simulink model "ADCS_orbiter"  (R2021b)
settings: Solver=VariableStepAuto  StartTime=0.0  StopTime=43200  FixedStep=0.01  MaxStep=1  RelTol=1e-8
values from neighbouring files (symbols this model uses):
  J = [Jx,0,0 ... (first row only)    [Data_detumbling.m]    (also in DisturbanceEvaluation.m = {J_NSO; J_SO}; Thruster_sizing_2.m = diag([12043.36, 15990.19, 8547.84]); main_orbiter.m = J_SO; main_orbiter_detumbling.m = J_SO)
  muE = (6.6743e-11)*(1.0802e20)    (= 7209578860)    [DisturbanceEvaluation.m]    (also in main_orbiter.m; main_orbiter_detumbling.m)
  muS = 3.7931187*1e16    (= 3.7931187e+16)    [DisturbanceEvaluation.m]    (also in main_orbiter.m; main_orbiter_detumbling.m)
  qbn0 = qrand./norm(qrand)    [main_orbiter.m]    (also in main_orbiter_detumbling.m)
  sigma_ARW = deg2rad(0.001)    [main_orbiter_detumbling.m]
  sigma_RRW = deg2rad(0.001)    [main_orbiter_detumbling.m]
  wb0 = 0.0001*rand(3, 1)    [main_orbiter.m]    (also in main_orbiter_detumbling.m = 0.1*rand(3, 1))
  Xpos = reshape(st_pos, [6, 1, L])    [main_orbiter.m]
undefined symbols (not defined in the file or in its folder): ICs, S
libraries: matrix_library x3, sublib_quat x1
settings Model: Creator=pietr  LastModifiedBy=26ele

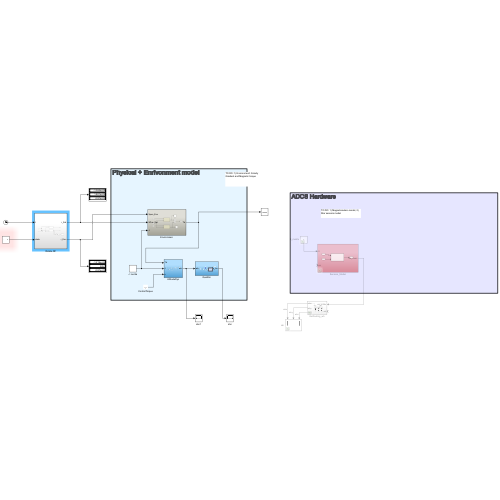
[thumbnail: Simulink's stored preview of the top-level diagram]
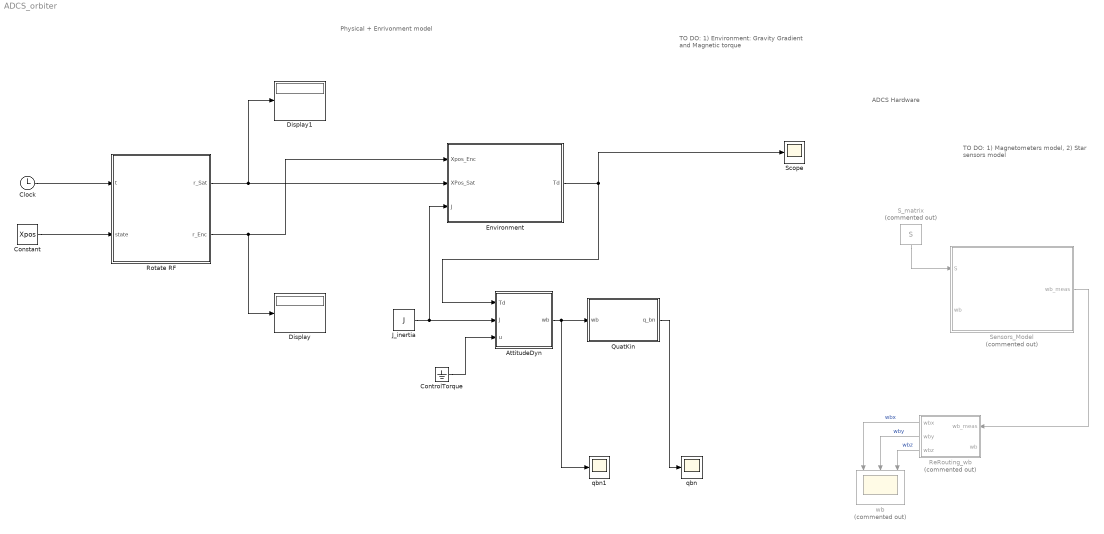
== system ADCS_orbiter ==
  note: TO DO: 1) Magnetometers model, 2) Star sensors model
  note: ADCS Hardware
  note: Physical + Enrivonment model
  note: TO DO: 1) Environment: Gravity Gradient and Magnetic torque
  AttitudeDyn : Subsystem
  Clock : Clock
      settings: Decimation=100
  Constant : Constant  Value=Xpos
  ControlTorque : Ground
  Display : Display
  Display1 : Display
  Environment : Subsystem
  J_inertia : Constant  Value=J  VectorParams1D=off
  QuatKin : Subsystem
  ReRouting_wb : Subsystem  Commented=on
  Rotate RF : Subsystem
  S_matrix : Constant  Commented=on  Value=S
  Scope : Scope
  Sensors_Model : Subsystem  Commented=on
  qbn : Scope
  qbn1 : Scope
  wb : Scope  Commented=on  NumInputPorts=3
  wires:
  AttitudeDyn/1(wb) -> qbn1/1, QuatKin/1(wb)
  QuatKin/1(q_bn) -> qbn/1
  ControlTorque/1 -> AttitudeDyn/3(u)
  S_matrix/1 -> Sensors_Model/1(S)
  Sensors_Model/1(wb_meas) -> ReRouting_wb/1(wb_meas)
  ReRouting_wb/1(wbx) -> wb/1  "wbx"
  ReRouting_wb/2(wby) -> wb/2  "wby"
  ReRouting_wb/3(wbz) -> wb/3  "wbz"
  J_inertia/1 -> AttitudeDyn/2(J), Environment/3(J)
  Environment/1(Td) -> AttitudeDyn/1(Td), Scope/1
  Rotate RF/2(r_Enc) -> Display/1, Environment/1(Xpos_Enc)
  Clock/1 -> Rotate RF/1(t)
  Constant/1 -> Rotate RF/2(state)
  Rotate RF/1(r_Sat) -> Display1/1, Environment/2(XPos_Sat)

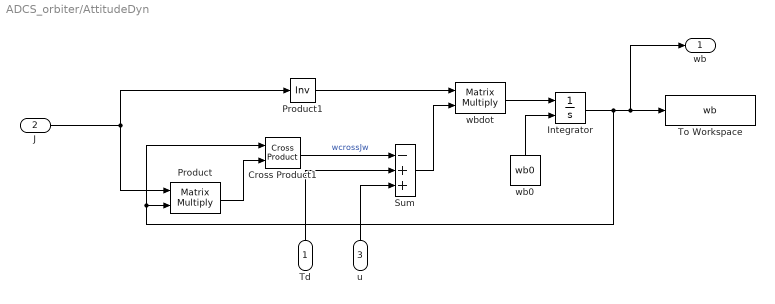
== system ADCS_orbiter/AttitudeDyn ==
  Td : Inport
  J : Inport  Port=2
  u : Inport  Port=3
  Cross Product1 : matrix_library/Cross Product
      settings: SourceProductBaseCode=SL
  Integrator : Integrator  InitialConditionSource=external
  Product : Product  Multiplication=Matrix(*)
  Product1 : Product  Inputs=/  Multiplication=Matrix(*)
  Sum : Sum  Inputs=-++
  To Workspace : ToWorkspace  VariableName=wb  SampleTime=-1
      settings: Save2DSignal=2-D array (concatenate along first dimension)
  wb0 : Constant  Value=wb0  VectorParams1D=off
  wbdot : Product  Multiplication=Matrix(*)
  wb : Outport
  wires:
  Integrator/1 -> wb/1, To Workspace/1, Product/2, Cross Product1/1
  Product/1 -> Cross Product1/2
  Cross Product1/1 -> Sum/1  "wcrossJw"
  J/1 -> Product1/1, Product/1
  wbdot/1 -> Integrator/1
  wb0/1 -> Integrator/2
  u/1 -> Sum/3
  Td/1 -> Sum/2
  Product1/1 -> wbdot/1
  Sum/1 -> wbdot/2

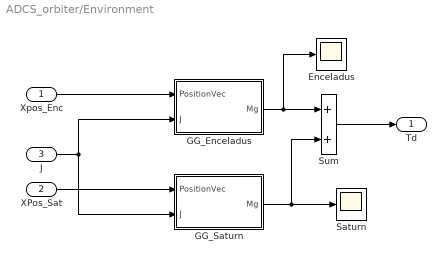
== system ADCS_orbiter/Environment ==
  Xpos_Enc : Inport
  XPos_Sat : Inport  Port=2
  J : Inport  Port=3
  Enceladus : Scope
  GG_Enceladus : Subsystem
  GG_Saturn : Subsystem
  Saturn : Scope
  Sum : Sum
  Td : Outport
  wires:
  Xpos_Enc/1 -> GG_Enceladus/1(PositionVec)
  J/1 -> GG_Saturn/2(J), GG_Enceladus/2(J)
  GG_Enceladus/1(Mg) -> Enceladus/1, Sum/1
  GG_Saturn/1(Mg) -> Saturn/1, Sum/2
  Sum/1 -> Td/1
  XPos_Sat/1 -> GG_Saturn/1(PositionVec)

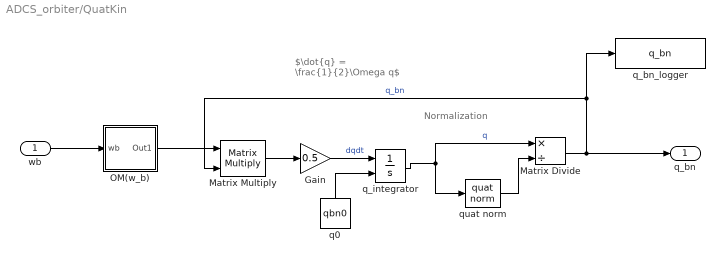
== system ADCS_orbiter/QuatKin ==
  note: $\dot{q} = \frac{1}{2}\Omega q$
  note: Normalization
  wb : Inport
  Gain : Gain  Gain=0.5
  Matrix Divide : Product  Inputs=*/
  Matrix Multiply : Product  Multiplication=Matrix(*)
  OM(w_b) : Subsystem
  q0 : Constant  Value=qbn0
  q_bn_logger : ToWorkspace  VariableName=q_bn  SampleTime=1
      settings: Save2DSignal=2-D array (concatenate along first dimension)
  q_integrator : Integrator  InitialConditionSource=external  InitialCondition=ICs.q_bn
  quat norm : sublib_quat/quat norm  SystemSampleTime=-1  VariantActivationTime=update diagram  Latency=0  AutoFrameSizeCalculation=off
      settings: SourceProductName=AOCS Team Blocks
  q_bn : Outport
  wires:
  q_integrator/1 -> quat norm/1, Matrix Divide/1  "q"
  OM(w_b)/1(Out1) -> Matrix Multiply/1
  quat norm/1 -> Matrix Divide/2
  Matrix Divide/1 -> q_bn/1, q_bn_logger/1, Matrix Multiply/2  "q_bn"
  Gain/1 -> q_integrator/1  "dqdt"
  Matrix Multiply/1 -> Gain/1
  wb/1 -> OM(w_b)/1(wb)
  q0/1 -> q_integrator/2

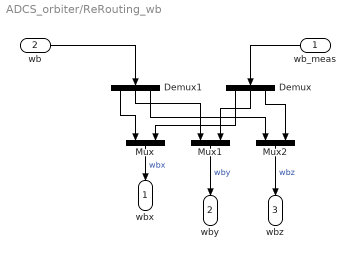
== system ADCS_orbiter/ReRouting_wb ==
  wb_meas : Inport
  wb : Inport  Port=2
  Demux : Demux  Outputs=3
  Demux1 : Demux  Outputs=3
  Mux : Mux  Inputs=2
  Mux1 : Mux  Inputs=2
  Mux2 : Mux  Inputs=2
  wbx : Outport
  wby : Outport  Port=2
  wbz : Outport  Port=3
  wires:
  Mux/1 -> wbx/1  "wbx"
  Demux1/3 -> Mux2/1
  Demux1/1 -> Mux/1
  Demux/1 -> Mux/2
  Demux1/2 -> Mux1/1
  Demux/3 -> Mux2/2
  Demux/2 -> Mux1/2
  wb_meas/1 -> Demux/1
  Mux1/1 -> wby/1  "wby"
  wb/1 -> Demux1/1
  Mux2/1 -> wbz/1  "wbz"

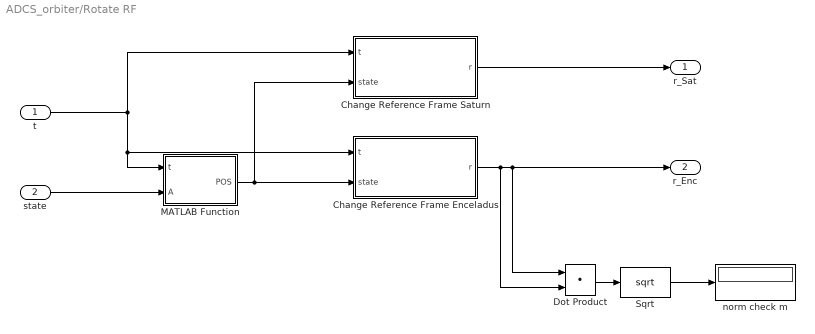
== system ADCS_orbiter/Rotate RF ==
  t : Inport
  state : Inport  Port=2
  Change Reference Frame Enceladus : MATLAB Function  TreatAsAtomicUnit=on
  Change Reference Frame Saturn : MATLAB Function  TreatAsAtomicUnit=on
  Dot Product : DotProduct  InputSameDT=on  OutDataTypeStr=Inherit: Inherit via internal rule
  MATLAB Function : MATLAB Function  TreatAsAtomicUnit=on
  Sqrt : Sqrt  SaturateOnIntegerOverflow=on
  norm check m : Display
  r_Sat : Outport
  r_Enc : Outport  Port=2
  wires:
  Sqrt/1 -> norm check m/1
  Change Reference Frame Enceladus/1(r) -> Dot Product/2, r_Enc/1, Dot Product/1
  t/1 -> Change Reference Frame Saturn/1(t), Change Reference Frame Enceladus/1(t), MATLAB Function/1(t)
  MATLAB Function/1(POS) -> Change Reference Frame Saturn/2(state), Change Reference Frame Enceladus/2(state)
  Dot Product/1 -> Sqrt/1
  state/1 -> MATLAB Function/2(A)
  Change Reference Frame Saturn/1(r) -> r_Sat/1

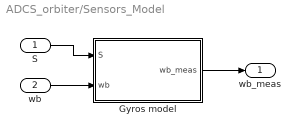
== system ADCS_orbiter/Sensors_Model ==
  S : Inport
  wb : Inport  Port=2
  Gyros model : Subsystem
  wb_meas : Outport
  wires:
  S/1 -> Gyros model/1(S)
  wb/1 -> Gyros model/2(wb)
  Gyros model/1(wb_meas) -> wb_meas/1

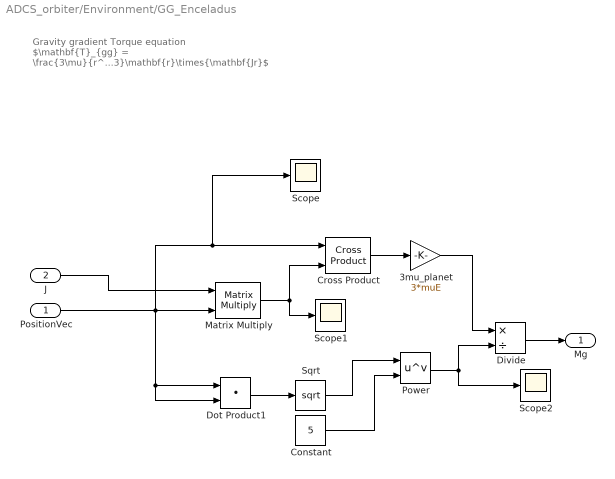
== system ADCS_orbiter/Environment/GG_Enceladus ==
  note: Gravity gradient Torque equation
      |
      | $\mathbf{T}_{gg} = \frac{3\mu}{r^3}\mathbf{r}\times{\mathbf{Jr}$
  PositionVec : Inport
  J : Inport  Port=2
  3mu_planet : Gain  Gain=3*muE
  Constant : Constant  Value=5
  Cross Product : matrix_library/Cross Product
      settings: SourceProductBaseCode=SL
  Divide : Product  Inputs=*/
  Dot Product1 : DotProduct  InputSameDT=on  OutDataTypeStr=Inherit: Inherit via internal rule
  Matrix Multiply : Product  Multiplication=Matrix(*)
  Power : Math  Operator=pow  SaturateOnIntegerOverflow=on
  Scope : Scope
  Scope1 : Scope
  Scope2 : Scope
  Sqrt : Sqrt  SaturateOnIntegerOverflow=on
  Mg : Outport
  wires:
  Constant/1 -> Power/2
  PositionVec/1 -> Matrix Multiply/2, Dot Product1/1, Dot Product1/2, Scope/1, Cross Product/1
  Matrix Multiply/1 -> Scope1/1, Cross Product/2
  J/1 -> Matrix Multiply/1
  3mu_planet/1 -> Divide/1
  Cross Product/1 -> 3mu_planet/1
  Power/1 -> Divide/2, Scope2/1
  Sqrt/1 -> Power/1
  Dot Product1/1 -> Sqrt/1
  Divide/1 -> Mg/1

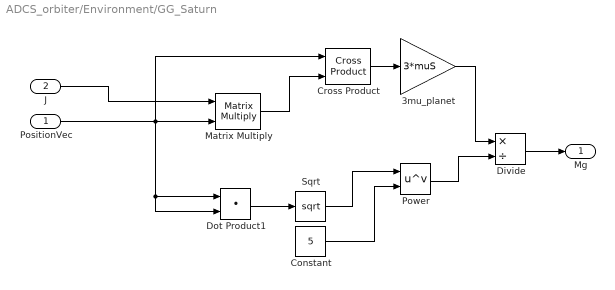
== system ADCS_orbiter/Environment/GG_Saturn ==
  PositionVec : Inport
  J : Inport  Port=2
  3mu_planet : Gain  Gain=3*muS
  Constant : Constant  Value=5
  Cross Product : matrix_library/Cross Product
      settings: SourceProductBaseCode=SL
  Divide : Product  Inputs=*/
  Dot Product1 : DotProduct  InputSameDT=on  OutDataTypeStr=Inherit: Inherit via internal rule
  Matrix Multiply : Product  Multiplication=Matrix(*)
  Power : Math  Operator=pow  SaturateOnIntegerOverflow=on
  Sqrt : Sqrt  SaturateOnIntegerOverflow=on
  Mg : Outport
  wires:
  Divide/1 -> Mg/1
  Dot Product1/1 -> Sqrt/1
  Sqrt/1 -> Power/1
  Power/1 -> Divide/2
  Cross Product/1 -> 3mu_planet/1
  3mu_planet/1 -> Divide/1
  J/1 -> Matrix Multiply/1
  Matrix Multiply/1 -> Cross Product/2
  PositionVec/1 -> Cross Product/1, Dot Product1/2, Dot Product1/1, Matrix Multiply/2
  Constant/1 -> Power/2

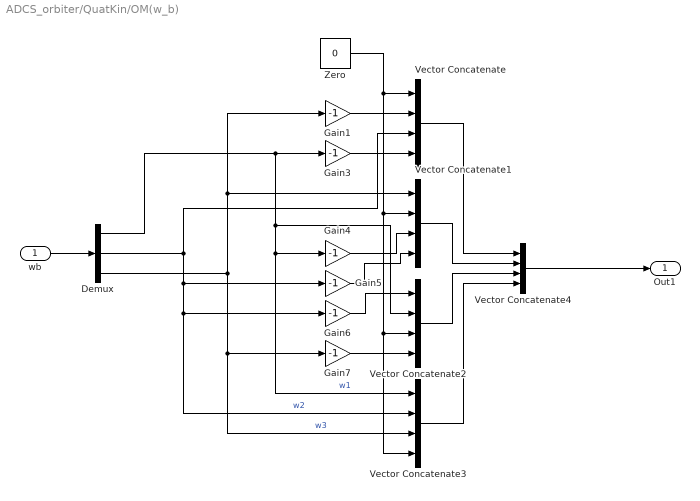
== system ADCS_orbiter/QuatKin/OM(w_b) ==
  wb : Inport
  Demux : Demux  Outputs=3
  Gain{1,3..7} (6 alike) : Gain  Gain=-1
  Vector Concatenate{,1..3} (4 alike) : Concatenate  NumInputs=4
  Vector Concatenate4 : Concatenate  NumInputs=4  Mode=Multidimensional array  ConcatenateDimension=2
  Zero : Constant  Value=0  OutDataTypeStr=Inherit: Inherit via back propagation
  Out1 : Outport
  wires:
  Demux/1 -> Vector Concatenate3/1, Gain4/1, Vector Concatenate2/2, Gain3/1  "w1"
  Vector Concatenate/1 -> Vector Concatenate4/1
  Zero/1 -> Vector Concatenate3/4, Vector Concatenate2/3, Vector Concatenate1/2, Vector Concatenate/1
  Gain7/1 -> Vector Concatenate2/4
  wb/1 -> Demux/1
  Demux/3 -> Vector Concatenate3/3, Gain7/1, Gain1/1, Vector Concatenate1/1  "w3"
  Gain5/1 -> Vector Concatenate1/4
  Gain3/1 -> Vector Concatenate/4
  Vector Concatenate4/1 -> Out1/1
  Vector Concatenate1/1 -> Vector Concatenate4/2
  Gain6/1 -> Vector Concatenate2/1
  Gain4/1 -> Vector Concatenate1/3
  Demux/2 -> Vector Concatenate3/2, Gain6/1, Gain5/1, Vector Concatenate/3  "w2"
  Vector Concatenate2/1 -> Vector Concatenate4/3
  Gain1/1 -> Vector Concatenate/2
  Vector Concatenate3/1 -> Vector Concatenate4/4

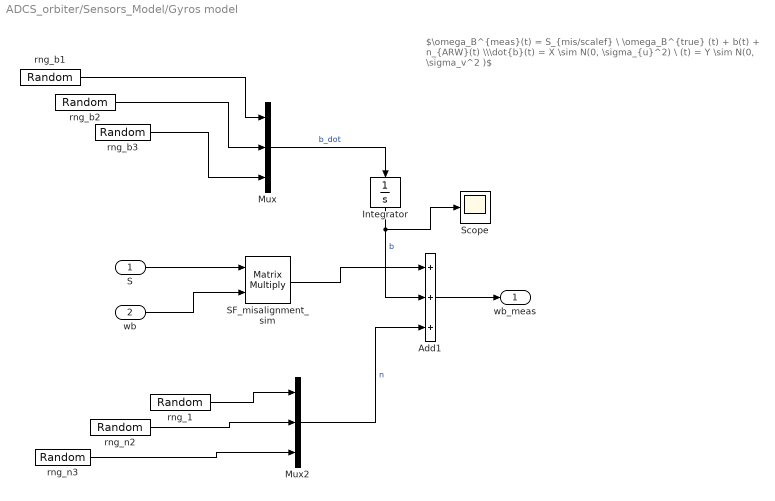
== system ADCS_orbiter/Sensors_Model/Gyros model ==
  note: $\omega_B^{meas}(t) = S_{mis/scalef} \ \omega_B^{true} (t) + b(t) + n_{ARW}(t) \\\dot{b}(t) = X \sim N(0, \sigma_{u}^2) \\n(t) = Y \sim N(0, \sigma_v^2 )$
  S : Inport
  wb : Inport  Port=2
  Add1 : Sum  Inputs=+++
  Integrator : Integrator  InitialCondition=[0; 0; 0]
  Mux : Mux  Inputs=3
  Mux2 : Mux  Inputs=3
  SF_misalignment_sim : Product  Multiplication=Matrix(*)
  Scope : Scope
  rng_1 : RandomNumber  Variance=sigma_ARW^2  Seed=6  SampleTime=0.1
  rng_b1 : RandomNumber  Variance=sigma_RRW^2  SampleTime=0.1
  rng_b2 : RandomNumber  Variance=sigma_RRW^2  Seed=3  SampleTime=0.1
  rng_b3 : RandomNumber  Variance=sigma_RRW^2  Seed=2  SampleTime=0.1
  rng_n2 : RandomNumber  Variance=sigma_ARW^2  Seed=7  SampleTime=0.1
  rng_n3 : RandomNumber  Variance=sigma_ARW^2  Seed=9  SampleTime=0.1
  wb_meas : Outport
  wires:
  Mux2/1 -> Add1/3  "n"
  Integrator/1 -> Scope/1, Add1/2  "b"
  Add1/1 -> wb_meas/1
  rng_b3/1 -> Mux/3
  rng_b1/1 -> Mux/1
  rng_1/1 -> Mux2/1
  wb/1 -> SF_misalignment_sim/2
  S/1 -> SF_misalignment_sim/1
  rng_b2/1 -> Mux/2
  rng_n2/1 -> Mux2/2
  Mux/1 -> Integrator/1  "b_dot"
  rng_n3/1 -> Mux2/3
  SF_misalignment_sim/1 -> Add1/1

== matlab function ADCS_orbiter/Rotate RF/MATLAB Function ==
  data: t input; POS output; A input
function POS = fcn(t, A)

t_ = floor(t+1);

if t_ >= 1

    POS = A(:, :, t_);
else
    POS = A(:,:, 1);
end

== matlab function ADCS_orbiter/Rotate RF/Change Reference Frame Saturn ==
  data: t input; r output; state input
function r = rotate_halo(t, state)

mu = 1.90095713928102*1e-7;      %[-] Saturn-Enceladus mass ratio

% Adimensionalization used for CRTBP Halo
DD = 238411468.296;              %[m]
TT=118760.57/(2*pi);             %[s]

t_ = floor(t+1)/TT;

% unpack state in Saturn-Enceladus rotating frame
xr = state(1);
yr = state(2);
zr = state(3);
vxr = state(4);
vyr = state(5);
vzr = state(6);

% From Saturn-Enceladus rotating frame to IAU_Saturn
X = (xr+mu)*cos(t_) - yr*sin(t_);
Y = (xr+mu)*sin(t_) + yr*cos(t_);
Z = zr;
VX = (vxr-yr)*cos(t_) - (vyr+xr+mu)*sin(t_);
VY = (vxr-yr)*sin(t_) + (vyr+xr+mu)*cos(t_);
VZ = vzr;

state_IAU_S = [X; Y; Z; VX; VY; VZ]; % IAU_Enceladus

% Dimensionalise again
r = state_IAU_S(1:3)*DD;                 % Dimensional in m

== matlab function ADCS_orbiter/Rotate RF/Change Reference Frame Enceladus ==
  data: t input; r output; state input
function r = rotate_halo(t, state)


mu = 1.90095713928102*1e-7;       %[-] Saturn-Enceladus mass ratio

% Adimensionalization used for CRTBP Halo
DD = 238411468.296;               %[m]
TT=118760.57/(2*pi);              %[s]

t_ = floor(t+1)/TT;

% unpack state in Saturn-Enceladus rotating frame
xr = state(1);
yr = state(2);
zr = state(3);
vxr = state(4);
vyr = state(5);
vzr = state(6);

% From Saturn-Enceladus rotating frame to IAU_Enceladus
X = (xr+mu-1)*cos(t_) - yr*sin(t_);
Y = (xr+mu-1)*sin(t_) + yr*cos(t_);
Z = zr;
VX = (vxr-yr)*cos(t_) - (vyr+xr+mu-1)*sin(t_);
VY = (vxr-yr)*sin(t_) + (vyr+xr+mu-1)*cos(t_);
VZ = vzr;

state_IAU_E = [X; Y; Z; VX; VY; VZ]; % IAU_Enceladus

% Dimensionalise again
r_IAU_E = state_IAU_E(1:3)*DD;                 % Dimensional in m

r = r_IAU_E;

% % DCM Matrix: rigid rotation around X 
% % (SAME REFERENCE USED FOR LANDING)
% A_rotx = [1  0  0
%           0  0  1
%           0 -1  0];
% 
% r = A_rotx*r_IAU_E;                            %[m]
